simulink model "robot_continu"  (R2015a)
settings: Solver=ode45  StartTime=0.0  StopTime=30  FixedStep=0.01  RelTol=1e-3
values from neighbouring files (symbols this model uses):
  K = -place(A,B,V)    [matrices.m]
undefined symbols (not defined in the file or in its folder): l
libraries: simulink x1
settings Model: Creator=gmartini  LastModifiedBy=root

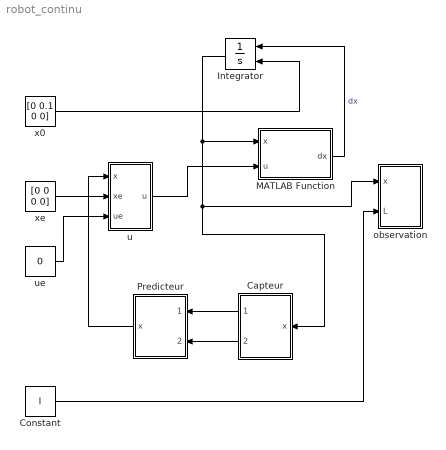
== system robot_continu ==
  Capteur : Subsystem
  Constant : Constant  Value=l
  Integrator : Integrator  InitialConditionSource=external
  MATLAB Function : MATLAB Function  TreatAsAtomicUnit=on
  Predicteur : Subsystem
  observation : Subsystem
  "u " : Subsystem
  ue : Constant  Value=0
  x0 : Constant  Value=[0 0.1 0 0]
  xe : Constant  Value=[0 0 0 0]
  wires:
  xe/1 -> "u "/2(xe)
  ue/1 -> "u "/3(ue)
  "u "/1(u) -> MATLAB Function/2(u)
  MATLAB Function/1(dx) -> Integrator/1  "dx"
  x0/1 -> Integrator/2
  Integrator/1 -> observation/1(x), Capteur/1(x), MATLAB Function/1(x)
  Capteur/1(nb_tour) -> Predicteur/1(nb_tour)
  Capteur/2(dpsi/dt) -> Predicteur/2(dpsi/dt)
  Predicteur/1(x) -> "u "/1(x)
  Constant/1 -> observation/2(L)

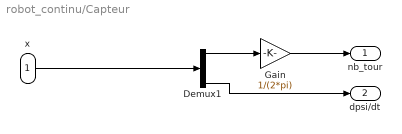
== system robot_continu/Capteur ==
  x : Inport
  Demux1 : Demux
  Gain : Gain  Gain=1/(2*pi)
  nb_tour : Outport
  dpsi/dt : Outport  Port=2
  wires:
  Gain/1 -> nb_tour/1
  Demux1/1 -> Gain/1
  Demux1/4 -> dpsi/dt/1
  x/1 -> Demux1/1

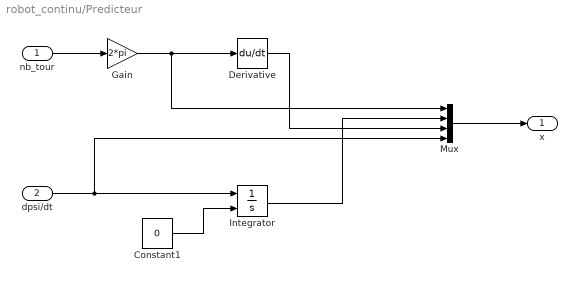
== system robot_continu/Predicteur ==
  nb_tour : Inport
  dpsi/dt : Inport  Port=2
  Constant1 : Constant  Value=0
  Derivative : Derivative
  Gain : Gain  Gain=2*pi
  Integrator : Integrator  InitialConditionSource=external
  Mux : Mux
  x : Outport
  wires:
  Integrator/1 -> Mux/2
  nb_tour/1 -> Gain/1
  Gain/1 -> Derivative/1, Mux/1
  dpsi/dt/1 -> Integrator/1, Mux/4
  Constant1/1 -> Integrator/2
  Derivative/1 -> Mux/3
  Mux/1 -> x/1

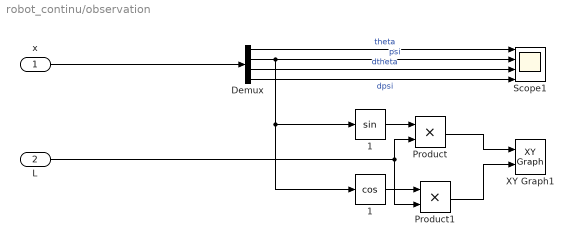
== system robot_continu/observation ==
  x : Inport
  L : Inport  Port=2
  " 1" : Trigonometry  Operator=cos
  " 1" : Trigonometry
  Demux : Demux
  Product : Product
  Product1 : Product
  Scope1 : Scope  NumInputPorts=4
      settings: YMin=130~-0.006~-8~-0.002  YMax=160~0.007~2~0.007
  XY Graph1 : simulink/Sinks/XY Graph  xmin=-0.1  xmax=0.1  ymin=-0.1  ymax=0.1  st=-1
  wires:
  Product/1 -> XY Graph1/1
  x/1 -> Demux/1
  L/1 -> Product1/2, Product/2
  Product1/1 -> XY Graph1/2
  " 1"/1 -> Product1/1
  " 1"/1 -> Product/1
  Demux/1 -> Scope1/1  "theta"
  Demux/3 -> Scope1/3  "dtheta"
  Demux/2 -> " 1"/1, " 1"/1, Scope1/2  "psi"
  Demux/4 -> Scope1/4  "dpsi"

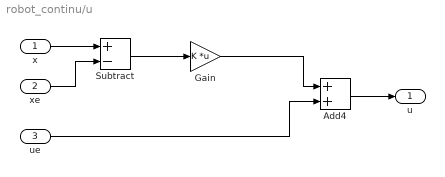
== system robot_continu/u  ==
  x : Inport
  xe : Inport  Port=2
  ue : Inport  Port=3
  Add4 : Sum
  Gain : Gain  Gain=K  Multiplication=Matrix(K*u)
  Subtract : Sum  Inputs=+-
  u : Outport
  wires:
  Add4/1 -> u/1
  ue/1 -> Add4/2
  xe/1 -> Subtract/2
  Gain/1 -> Add4/1
  x/1 -> Subtract/1
  Subtract/1 -> Gain/1

== matlab function robot_continu/MATLAB Function ==
  data: x input; u input; dx output
function dx = fonction( x, u)
%   Dynamic equations of motion of the segway on an axis.
%   Inputs: - x = [theta psi dtheta dpsi]
%               theta: average angle of the wheels      [rad]
%               psi: body pitch angle                   [rad]
%               dtheta: average velocity of the wheels  [rad/s]
%               dpsi: body pitch velocity               [rad/s]
%          - u: DC motor voltage (same value for both motors) [V]

    % State
    psi = x(2);
    dtheta = x(3);
    dpsi = x(4);

    % Parameters
    
    g = 9.81;           % gravity acceleration [m/sec^2]
    m = 0.03;           % wheel weight [kg]
    R = 0.04;           % wheel radius [m]
    Jw = m*R^2/2;       % wheel inertia moment [kg*m^2]
    M = 0.6;            % body weight [kg]
    H = 0.144;          % body height [m]
    L = H/2;            % distance of the center of mass from the wheel axle [m]
    Jpsi = M*L^2/3;     % body pitch inertia [kgm^2]
    Jm = 1e-5;          % DC motor inertia moment [kgm^2]
    Rm = 6.69;          % DC motor resistance [Ohm]
    Kb = 0.468;         % DC motor back EMF constant [Vsec/rad]
    Kt = 0.317;         % DC motor torque constant [Nm/A]
    n = 1;              % gear ratio
    fm = 0.0022;        % friction coefficient between body and DC motor
    fw = 0;             % friction coefficient between wheel and floor
    
    % Equations of motion
    c1 = (2*m+M)*R^2 + 2*Jw + 2*n^2*Jm;
    c2 = M*L*R*cos(psi) - 2*n^2*Jm;
    c3 = -M*L*R*dpsi^2*sin(psi);
    c4 = M*L^2 + Jpsi + 2*n^2*Jm;
    c5 = -M*g*L*sin(psi);

    alpha = Kt/Rm;
    beta = Kt*Kb/Rm + fm;

    Ftheta = alpha*(2*u) - 2*(beta+fw)*dtheta + 2*beta*dpsi;
    Fpsi = -alpha*(2*u) + 2*beta*dtheta - 2*beta*dpsi;

    ddtheta = (c4*c3 - c2*c5 + c4*Ftheta - c2*Fpsi)/(c4*c1 - c2^2);
    ddpsi = (Fpsi- c2*ddtheta - c5)/c4;
    dx = [dtheta dpsi ddtheta ddpsi]';

end

% Matrices of the linearized system
% E = [(2*m+M)*R^2+2*Jw+2*Jm   M*L*R-2*Jm; M*L*R-2*Jm   M*L^2+Jpsi+2*Jm];
% detE = det(E);

% alpha = Kt/Rm;
% beta = Kt*Kb/Rm + fm;

% A32 = -M*g*L*E(1,2)/detE;
% A42 = M*g*L*E(1,1)/detE;
% A33 = -(beta*E(2,2)+2*beta*E(1,2))/detE;
% A43 = (beta*E(1,2)+2*beta*E(1,1))/detE;
% A34 = beta*(E(2,2)+2*E(1,2))/detE;
% A44 = -beta*(E(1,2)+2*E(1,1))/detE;

% B3 = alpha*(E(2,2)/2+E(1,2))/detE;
% B4 = -alpha*(E(1,2)/2+E(1,1))/detE;

% A = [0 0 1 0;0 0 0 1; 0 A32 A33 A34; 0 A42 A43 A44];
% B = [0 0 2*B3 2*B4];
